simulink model "real_time_test"  (R2021a)
settings: Solver=FixedStepAuto  StartTime=0.0  StopTime=10  RelTol=1e-3
libraries: dspvision x3, visionsources x2
settings Model: Creator=Owner  LastModifiedBy=Owner
settings SolverCC: ConcurrentTasks=on  PositivePriorityOrder=on
settings OptimizationCC: BlockReduction=off  OptimizeBlockIOStorage=off
settings DebuggingCC: TasksWithSamePriorityMsg=none
settings HardwareCC: ProdBitPerLong=64  ProdLongLongMode=on  ProdHWDeviceType=Intel->x86-64 (Linux 64)
settings RTWCC: Description=Simulink Real-Time  SystemTargetFile=slrealtime.tlc  TemplateMakefile=slrealtime_default_tmf  Toolchain=Simulink Real-Time Toolchain  BuildConfiguration=Faster Runs  CodeExecutionProfiling=on  TargetLang=C++

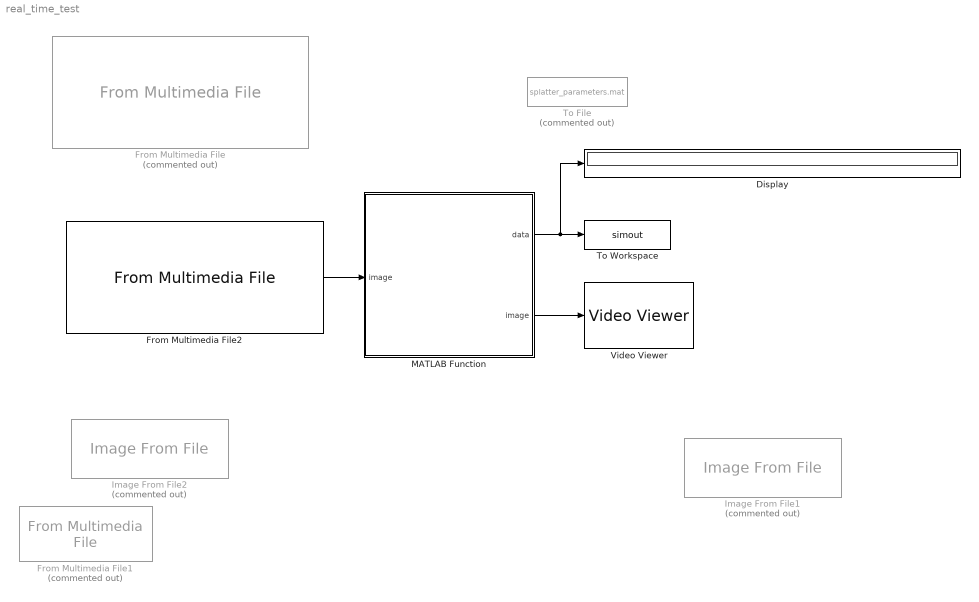
== system real_time_test ==
  Display : Display
  From Multimedia File : dspvision/From Multimedia File  Commented=on  inputFilename=C:\Users\Owner\Downloads\FILR_edit.mp4  readRange=[1 Inf]  loop=on  numPlays=inf  outputStreams=Video only  videoDataType=single  audioDataType=int16  inheritSampleTime=on  userDefinedSampleTime=1/30  noAudioOutput=off  isIntensityVideo=off  fourcc=RGB  colorVideoFormat=One multidimensional signal  outputEOF=off  dataOrg=Column-major  audioFrameSize=1024  computeAudioFrameSize=off  outSamplingMode=Sample based
  From Multimedia File1 : dspvision/From Multimedia File  Commented=on  inputFilename=C:\Users\Owner\OneDrive\Documents\Python Scripts\Senior-Design-Project-EMCH427-002-Team-4-Downey\Software\images\test_vid.mov  readRange=[1 Inf]  loop=on  numPlays=inf  outputStreams=Video only  videoDataType=single  audioDataType=int16  inheritSampleTime=on  userDefinedSampleTime=1/30  noAudioOutput=off  isIntensityVideo=off  fourcc=RGB  colorVideoFormat=One multidimensional signal  outputEOF=off  dataOrg=Column-major  audioFrameSize=1024  computeAudioFrameSize=off  outSamplingMode=Sample based
  From Multimedia File2 : dspvision/From Multimedia File  inputFilename=C:\Users\Owner\Downloads\smallest_125w150mms_powder_v3.avi  readRange=[1 Inf]  loop=on  numPlays=inf  outputStreams=Video only  videoDataType=single  audioDataType=int16  inheritSampleTime=on  userDefinedSampleTime=1/30  noAudioOutput=off  isIntensityVideo=off  fourcc=RGB  colorVideoFormat=One multidimensional signal  outputEOF=off  dataOrg=Column-major  audioFrameSize=1024  computeAudioFrameSize=off  outSamplingMode=Sample based
  Image From File1 : visionsources/Image From File  Tag=vipblks_nd  Commented=on  FileName=C:\Users\Owner\OneDrive\Documents\Python Scripts\Senior-Design-Project-EMCH427-002-Team-4-Downey\Software\images\FILR\FILR_edit11.jpg  Ts=inf  imagePorts=One multidimensional signal  OutPortLabels=R|G|B  ImageDataType=Inherit from input image  sdImageDataType=uint(8)  Signed=on  WordLength=16  FractionLengthMode=User-defined  FractionLength=15
  Image From File2 : visionsources/Image From File  Tag=vipblks_nd  Commented=on  FileName=C:\Users\Owner\OneDrive\Documents\Python Scripts\Senior-Design-Project-EMCH427-002-Team-4-Downey\Software\images\0.png  Ts=inf  imagePorts=One multidimensional signal  OutPortLabels=R|G|B  ImageDataType=Inherit from input image  sdImageDataType=uint(8)  Signed=on  WordLength=16  FractionLengthMode=User-defined  FractionLength=15
  MATLAB Function : MATLAB Function  TreatAsAtomicUnit=on
  To File : ToFile  Commented=on  Filename=splatter_parameters.mat  SaveFormat=Timeseries
  To Workspace : ToWorkspace  VariableName=simout  SaveFormat=Structure With Time  SampleTime=-1
      settings: Save2DSignal=2-D array (concatenate along first dimension)
  Video Viewer : VideoViewer  FigPos=[-890 783 418 304]
  wires:
  MATLAB Function/1(data) -> Display/1, To Workspace/1
  MATLAB Function/2(image) -> Video Viewer/1
  From Multimedia File2/1 -> MATLAB Function/1("image ")

== matlab function real_time_test/MATLAB Function ==
  data: data output; image input; image output
function [data, image] = ProcessFrames(image)
    data = zeros(1,5);

    gray = rgb2gray(image);

%     copy = imgaussfilt(gray,0.1); %standard deviation of 2

%     copy = 215 < gray; %thresh
    copy = imbinarize(gray,0.85);
    
    copy(2:6,2:9) = 1;
    copy(:,1) = 0;
    copy(:,end) = 0;
    copy(1,:) = 0;
    copy(end,:) = 0;
    
    %     SE = strel('line',1,1);
    %     copy = imerode(copy,SE);
    PixelList = zeros(2,0);
    stats = regionprops(copy, 'Area','Centroid', 'EquivDiameter', 'PixelList');
    idx = 0;
    brightness = 0;
    for i = 1:length(stats)
        
        if stats(i).Area >= 10
            PixelList = [PixelList stats(i).PixelList'];
            brightness = 1+brightness;
            
            if stats(i).Area > data(3)
                data(3) = stats(i).Area;
                idx = i;
            end
            
        end
        
    end


    
    data(1) = ceil(stats(idx).Centroid(1));     %X
    data(2) = ceil(stats(idx).Centroid(2));     %Y
    %data(3) =                                  %Area
    data(4) = stats(idx).EquivDiameter(end)/2;  %Radius
    data(5) = brightness;                              %Brightness
    
    %     brightness = zeros(length(PixelList(:,1)),1);
    %     % 
    %     for idx = 1:1:length(PixelList(:,1))
    %         pixel = PixelList(idx,:);
    %         lumen = gray(pixel(1), pixel(2));
    %         brightness(idx) = lumen;
    %     end
    %     brightness = round(mean(brightness));

    % dilate = imdilate(erode,SE);
    % imshow(erode)
    % imshow(copy)
    %     montage({image,gray,gaus,thresh,erode})
    

    %     horz = length(image(1,:))/3;
    %     vert = length(image(:,1));
    %     text_str = cell(5,1);
    %     text_str{1} = ['X: ' num2str(centroid(1),'%0.2f')];
    %     text_str{2} = ['Y: ' num2str(centroid(2),'%0.2f')];
    %     text_str{3} = ['Area: ' num2str(max_area,'%0.2f')];
    %     text_str{4} = ['Radius: ' num2str(radius,'%0.2f')];
    %     text_str{5} = ['Brightness: ' num2str(brightness,'%0.2f')];
    %     
    %     positions = [0 vert-vert/8; horz/5 vert-vert/8; 0 vert-vert/8-30; horz-horz/3 vert-vert/8-30; horz-horz/3 vert-vert/8];

    %     image = insertText(image, positions, text_str,'FontSize',9,'BoxColor',...
    %         [255 0 0],'BoxOpacity',0.4,'TextColor',[255 255 255]);
    
%     [B,~]= bwboundaries(copy);
%     for k = 1:length(B{1,1}(:,2))
%         image(B{1,1}(k,1) ,B{1,1}(k,2),:) = [255 0 0];
%         
%         image(B{1,1}(k,1) ,B{1,1}(k,2)+1,:) = [255 0 0];
%         image(B{1,1}(k,1) ,B{1,1}(k,2)-1,:) = [255 0 0];
%         image(B{1,1}(k,1)+1 ,B{1,1}(k,2),:) = [255 0 0];
%         image(B{1,1}(k,1)-1 ,B{1,1}(k,2),:) = [255 0 0];
%         
%     end
    
    
    PixelList = PixelList';
    for k = 1:1:length(PixelList(:,1))
            pixel = PixelList(k,:);
%             copy(pixel(2), pixel(1));

            if copy(pixel(2)+1,pixel(1)) == 0
                image(pixel(2)+1,pixel(1),:) = [255 0 0];
                image(pixel(2),pixel(1),:) = [255 0 0];
            end

            if copy(pixel(2)-1,pixel(1)) == 0
                image(pixel(2)-1,pixel(1),:) = [255 0 0];
                image(pixel(2),pixel(1),:) = [255 0 0];
            end

            if copy(pixel(2),pixel(1)+1) == 0
                image(pixel(2),pixel(1)+1,:) = [255 0 0];
                image(pixel(2),pixel(1),:) = [255 0 0];
            end

            if copy(pixel(2),pixel(1)-1) == 0
                image(pixel(2),pixel(1)-1,:) = [255 0 0];
                image(pixel(2),pixel(1),:) = [255 0 0];
            end

    end

    
end
